simulink model "Task2_3"  (R2022a)
settings: Solver=FixedStepAuto  StartTime=0.0  StopTime=20  FixedStep=0.0001  RelTol=1e-3
undefined symbols (not defined in the file): A, B, C, D1, D2, Dblock, x1
settings Model: Creator=Family  LastModifiedBy=Family

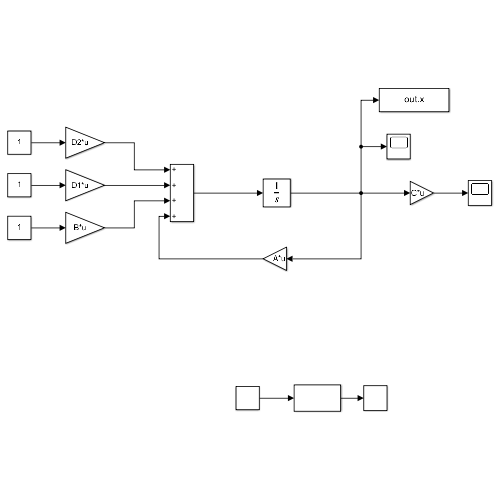
[thumbnail: Simulink's stored preview of the top-level diagram]
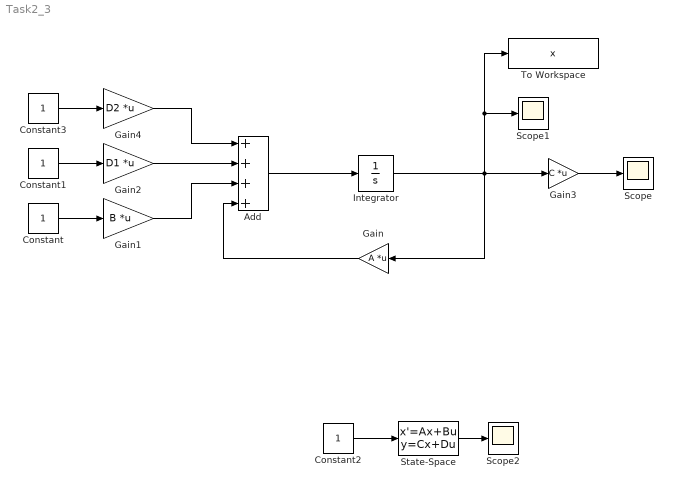
== system Task2_3 ==
  Add : Sum  Inputs=++++
  Constant{,1..3} (4 alike) : Constant
  Gain : Gain  Gain=A  Multiplication=Matrix(K*u)
  Gain1 : Gain  Gain=B  Multiplication=Matrix(K*u)
  Gain2 : Gain  Gain=D1  Multiplication=Matrix(K*u)
  Gain3 : Gain  Gain=C  Multiplication=Matrix(K*u)
  Gain4 : Gain  Gain=D2  Multiplication=Matrix(K*u)
  Integrator : Integrator  InitialCondition=x1
  Scope : Scope
  Scope1 : Scope
  Scope2 : Scope
  State-Space : StateSpace  A=A  B=B  C=C  D=Dblock  InitialCondition=0
  To Workspace : ToWorkspace  VariableName=x  SaveFormat=Timeseries  SampleTime=-1
  wires:
  Integrator/1 -> Gain/1, Gain3/1, To Workspace/1, Scope1/1
  Add/1 -> Integrator/1
  Gain/1 -> Add/4
  Gain1/1 -> Add/3
  Constant/1 -> Gain1/1
  Constant1/1 -> Gain2/1
  Gain3/1 -> Scope/1
  State-Space/1 -> Scope2/1
  Constant2/1 -> State-Space/1
  Constant3/1 -> Gain4/1
  Gain4/1 -> Add/1
  Gain2/1 -> Add/2
